simulink model "LQI_Giuse"  (R2024b)
settings: Solver=VariableStepAuto  StartTime=0.0  StopTime=10.0  RelTol=1e-3
values from neighbouring files (symbols this model uses):
  A_p = [0, 1; (2*km*(u_e^2))/(m*((l - x1_e - (2*r)))^3) 0]    [LQI_Giuse_code.m]
  B_p = [0; (2*km*u_e)/(m*((l - x1_e - (2*r)))^2)]    [LQI_Giuse_code.m]
  C_p = [1, 0]    [LQI_Giuse_code.m]
  D_p = 0    [LQI_Giuse_code.m]
  g = 9.81    [LQI_Giuse_code.m]    (also in SS_model_LQ.m)
  Ki_i = Ki_p/Ti    [LQI_Giuse_code.m]    (also in SS_model_LQ.m = 1650.02619)
  Ki_p = sqrt(R_tot^2 + (wc*Lc)^2) / ( Kg * sqrt(1 + 1/(wc^2 * Ti^2)) )    [LQI_Giuse_code.m]
  km = 6.5308e-5    (= 6.5308e-05)    [LQI_Giuse_code.m]    (also in SS_model_LQ.m)
  l = 0.0394    [LQI_Giuse_code.m]    (also in SS_model_LQ.m)
  Lc = 412.5e-3    (= 0.4125)    [LQI_Giuse_code.m]
  m = 0.068    [LQI_Giuse_code.m]    (also in SS_model_LQ.m)
  r = 1.27e-2    (= 0.0127)    [LQI_Giuse_code.m]    (also in SS_model_LQ.m)
  R_tot = (Rc + Rs)* Rcal    (= 9.35)    [LQI_Giuse_code.m]
  Rn = 1e-4    (= 0.0001)    [LQI_Giuse_code.m]
  u_e = (((g*m)/km)^(1/2))*(l - x1_e - (2*r))    (= 0.70746312484)    [LQI_Giuse_code.m]
  x1_e = 0.007    [LQI_Giuse_code.m]
undefined symbols (not defined in the file or in its folder): Continuous, K, Time
libraries: slpidlib x1, ctrlSharedLib x1
settings Model: Creator=gsacc  LastModifiedBy=gsacc

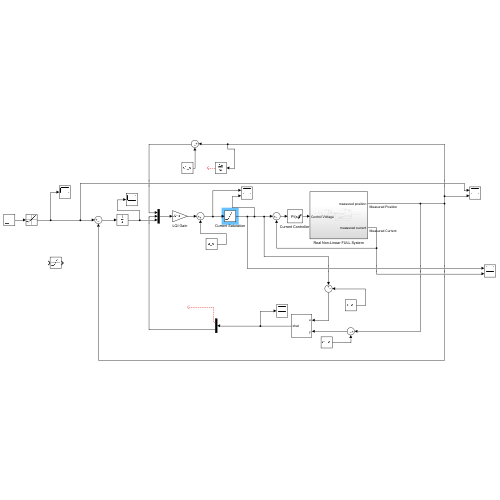
[thumbnail: Simulink's stored preview of the top-level diagram]
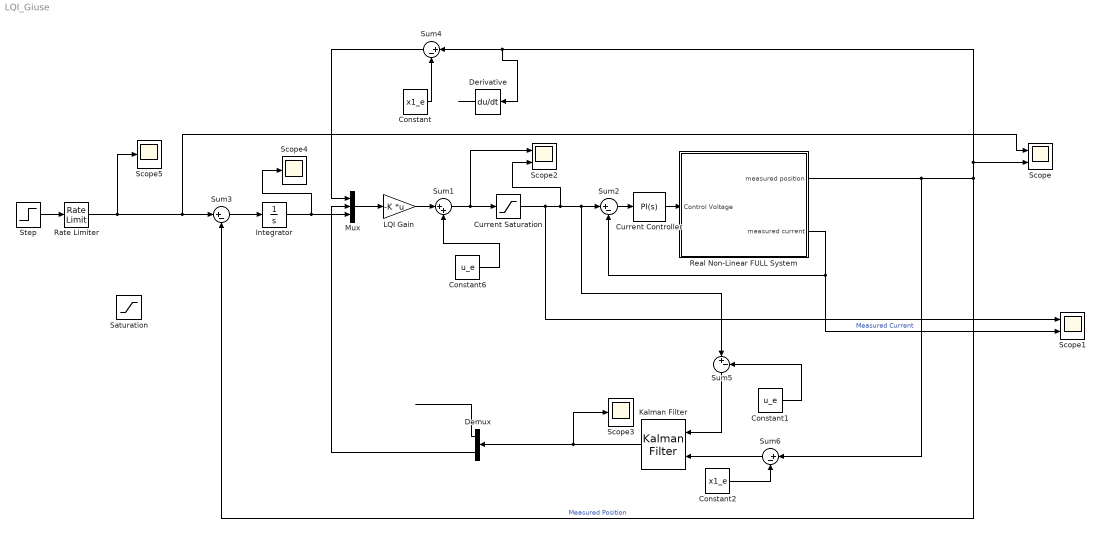
== system LQI_Giuse ==
  Constant : Constant  Value=x1_e
  Constant1 : Constant  Value=u_e
  Constant2 : Constant  Value=x1_e
  Constant6 : Constant  Value=u_e
  "Current Controller " : slpidlib/PID Controller  Controller=PI  Form=Parallel  TimeDomain=Continuous-time  UseExternalTs=off  SampleTime=-1  IntegratorMethod=Forward Euler  FilterMethod=Forward Euler  ControllerParametersSource=internal  P=Ki_p  I=Ki_i  UseKiTs=off  D=0  UseExternalDerivativeSource=off  N=0  UseFilter=on  TunerSelectOption=Transfer Function Based (PID Tuner App)  InitialConditionSource=internal  InitialConditionForIntegrator=0  InitialConditionForFilter=0  DifferentiatorICPrevScaledInput=0  ExternalReset=none  TrackingMode=off  Kt=1  LimitOutput=on  SatLimitsSource=internal  UpperSaturationLimit=8  LowerSaturationLimit=-8  LinearizeAsGain=off  AntiWindupMode=back-calculation  Kb=1  LimitIntegrator=off  UpperIntegratorSaturationLimit=inf  LowerIntegratorSaturationLimit=-inf  POutMin=[]  POutMax=[]  IOutMin=[]  IOutMax=[]  DOutMin=[]  DOutMax=[]  NOutMin=[]  NOutMax=[]  SumOutMin=[]  SumOutMax=[]  SaturationOutMin=[]  SaturationOutMax=[]  PParamMin=[]  PParamMax=[]  IParamMin=[]  IParamMax=[]  DParamMin=[]  DParamMax=[]  NParamMin=[]  NParamMax=[]  KbParamMin=[]  KbParamMax=[]  KtParamMin=[]  KtParamMax=[]  KbOutMin=[]  KbOutMax=[]  KtOutMin=[]  KtOutMax=[]  IntegratorOutMin=[]  IntegratorOutMax=[]  FilterOutMin=[]  FilterOutMax=[]  SumI1OutMin=[]  SumI1OutMax=[]  SumI2OutMin=[]  SumI2OutMax=[]  SumI3OutMin=[]  SumI3OutMax=[]  SumI4OutMin=[]  SumI4OutMax=[]  SumDOutMin=[]  SumDOutMax=[]  DifferentiatorOutMin=[]  DifferentiatorOutMax=[]  FilterDiffOutCoefMin=[]  FilterDiffOutCoefMax=[]  ReciprocalOutMin=[]  ReciprocalOutMax=[]  SumDenOutMin=[]  SumDenOutMax=[]  SumNumOutMin=[]  SumNumOutMax=[]  DivideOutMin=[]  DivideOutMax=[]  UdiffTsProdOutMin=[]  UdiffTsProdOutMax=[]  NTsProdOutMin=[]  NTsProdOutMax=[]  UintegralTsProdOutMin=[]  UintegralTsProdOutMax=[]  UngainTsProdOutMin=[]  UngainTsProdOutMax=[]  ClampingZeroOutDataTypeStr=Inherit: Inherit via back propagation  ClampingZeroOutMin=[]  ClampingZeroOutMax=[]  FilterDenConstantOutDataTypeStr=Inherit: Inherit via back propagation  FilterDenConstantOutMin=[]  FilterDenConstantOutMax=[]  PCopyOutDataTypeStr=Inherit: Inherit via back propagation  PCopyOutMin=[]  PCopyOutMax=[]  NCopyOutDataTypeStr=Inherit: Inherit via back propagation  NCopyOutMin=[]  NCopyOutMax=[]  IntegratorContinuousStateAttributes=''  IntegratorStateMustResolveToSignalObject=off  IntegratorRTWStateStorageClass=Auto  FilterContinuousStateAttributes=''  FilterStateMustResolveToSignalObject=off  FilterRTWStateStorageClass=Auto  ParallelPVariant=InternalParameters  IdealPVariant=Disabled  IVariant=InternalParameters  DVariant=Disabled  IntegratorVariant=Continuous  SatVariant=Enabled  AWVariant=BackCalculation  PCopyVariant=Disabled  TRVariant=Disabled  FdbkBlocksVariant=Forward  IdealPFdbkVariant=Disabled  SatFdbkVariant=Disabled  DerivativeFilterVariant=Disabled  NVariant=Disabled  NCopyVariant=Disabled_SignalSpec  FilterICVariant=Disabled  IntegratorICVariant=InternalICs  ExternalResetVariant=Disabled  TRSumVariant=Passthrough  SumFdbkVariant=Disabled  SumVariant=Sum_PI  TsampFilterVariant=InternalTs  TsampNgainVariant=Passthrough  TsampIntegralVariant=Disabled_SignalSpec  ExternalSaturationOutDataTypeStr=Inherit: Same as second input  DerivativeSourceVariant=Disabled  PreIntVariant=InternalPreInt
  Current Saturation : Saturate  UpperLimit=3  LowerLimit=-3
  Demux : Demux  Outputs=2
  Derivative : Derivative
  Integrator : Integrator
  Kalman Filter : ctrlSharedLib/Kalman Filter  TimeDomain=Continuous-Time  UseCurrentEstimator=on  ModelSource=Individual A, B, C, D matrices  ModelSourceVariable=ss(0.95,1,1,0,1)  A=A_p  B=B_p  C=C_p  D=D_p  NumberOfStates=1  NumberOfInputs=1  NumberOfOutputs=1  InitialEstimateSource=Dialog  X0=0  P0=10  UseK=off  UseGH=off  NumberOfProcessNoiseInputs=1  G=1  TimeInvariantG=on  H=0  TimeInvariantH=on  Q=Qn  TimeInvariantQ=on  R=Rn  TimeInvariantR=on  N=0  TimeInvariantN=on  AddInputPort=on  AddEnablePort=off  OutputEstimatedY=off  OutputP=off  Ts=-1
  LQI Gain : Gain  Gain=-K  Multiplication=Matrix(K*u)
  Mux : Mux  Inputs=3
  Rate Limiter : RateLimiter  RisingSlewLimit=0.007/0.5  SampleTimeMode=inherited
  Real Non-Linear FULL System : Subsystem
  Saturation : Saturate
  Scope : Scope  NumInputPorts=2
  Scope1 : Scope  NumInputPorts=2
  Scope2 : Scope  NumInputPorts=2
  Scope3 : Scope
  Scope4 : Scope
  Scope5 : Scope
  Step : Step  Time=0.1  After=x1_e  SampleTime=0
  Sum1 : Sum  Inputs=|++
  Sum{2..6} (5 alike) : Sum  Inputs=|+-
  wires:
  "Current Controller "/1 -> Real Non-Linear FULL System/1(Control Voltage)
  Real Non-Linear FULL System/1(measured position) -> Sum6/1, Sum4/1, Derivative/1, Scope/2, Sum3/2  "Measured Position"
  Sum1/1 -> Scope2/1, Current Saturation/1
  LQI Gain/1 -> Sum1/1
  Constant6/1 -> Sum1/2
  Current Saturation/1 -> Scope1/1, Scope2/2, Sum5/1, Sum2/1
  Sum2/1 -> "Current Controller "/1
  Real Non-Linear FULL System/2(measured current) -> Sum2/2, Scope1/2  "Measured Current"
  Mux/1 -> LQI Gain/1
  Step/1 -> Rate Limiter/1
  Derivative/1 -> ?
  Constant/1 -> Sum4/2
  Sum4/1 -> Mux/1
  Kalman Filter/1 -> Scope3/1, Demux/1
  Demux/1 -> ?
  Integrator/1 -> Scope4/1, Mux/3
  Demux/2 -> Mux/2
  Constant2/1 -> Sum6/2
  Sum6/1 -> Kalman Filter/2
  Sum5/1 -> Kalman Filter/1
  Constant1/1 -> Sum5/2
  Sum3/1 -> Integrator/1
  Rate Limiter/1 -> Scope/1, Sum3/1, Scope5/1

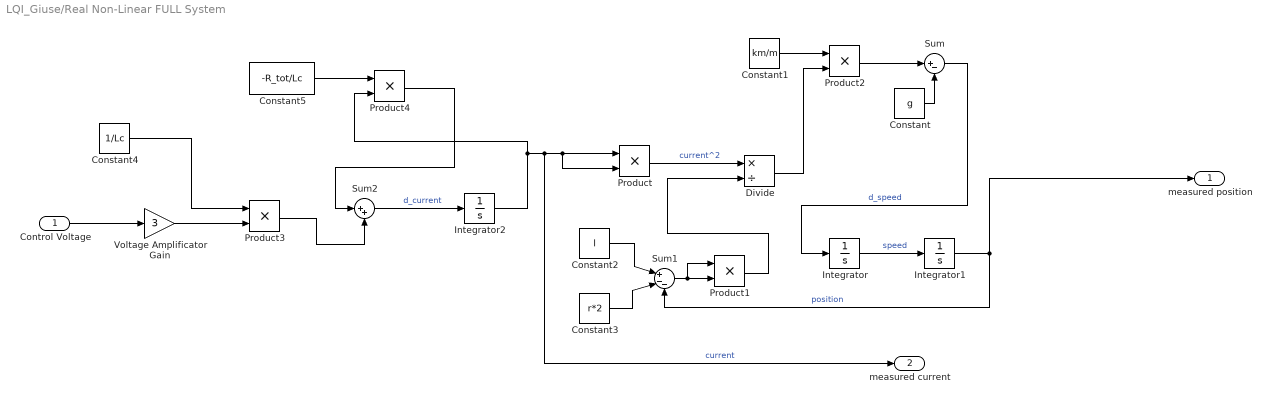
== system LQI_Giuse/Real Non-Linear FULL System ==
  Control Voltage : Inport
  Constant : Constant  Value=g
  Constant1 : Constant  Value=km/m
  Constant2 : Constant  Value=l
  Constant3 : Constant  Value=r*2
  Constant4 : Constant  Value=1/Lc
  Constant5 : Constant  Value=-R_tot/Lc
  Divide : Product  Inputs=*/
  Integrator : Integrator
  Integrator1 : Integrator  LimitOutput=on  UpperSaturationLimit=0.014  LowerSaturationLimit=0
  Integrator2 : Integrator
  Product{,1..4} (5 alike) : Product
  Sum : Sum  Inputs=|+-
  Sum1 : Sum  Inputs=|+--
  Sum2 : Sum  Inputs=|++
  Voltage Amplificator Gain : Gain  Gain=3
  measured position : Outport
  measured current : Outport  Port=2
  wires:
  Integrator/1 -> Integrator1/1  "speed"
  Integrator1/1 -> measured position/1, Sum1/3  "position"
  Constant2/1 -> Sum1/1
  Constant3/1 -> Sum1/2
  Sum1/1 -> Product1/2, Product1/1
  Product/1 -> Divide/1  "current^2"
  Product1/1 -> Divide/2
  Constant/1 -> Sum/2
  Constant1/1 -> Product2/1
  Divide/1 -> Product2/2
  Product2/1 -> Sum/1
  Sum/1 -> Integrator/1  "d_speed"
  Constant4/1 -> Product3/1
  Control Voltage/1 -> Voltage Amplificator Gain/1
  Product3/1 -> Sum2/2
  Integrator2/1 -> Product/1, Product/2, measured current/1, Product4/2  "current"
  Sum2/1 -> Integrator2/1  "d_current"
  Constant5/1 -> Product4/1
  Product4/1 -> Sum2/1
  Voltage Amplificator Gain/1 -> Product3/2
